simulink model "a_T_vector"  (R2016b)
settings: Solver=VariableStepAuto  StartTime=0.0  StopTime=tgoest  RelTol=1e-3
values from neighbouring files (symbols this model uses):
  m0 = 58000    [E_Guidance_Modular.m]    (also in E_Guidance_Wong.m; E_Guidance_advanced.m; E_Guidance_advanced_hybrid.m; E_Guidance_advanced_thrust_optimization.m)
  mu = 4.282828185603917*10^13    (= 4.2828281856e+13)    [E_Guidance_Modular.m]    (also in E_Guidance_Wong.m; E_Guidance_advanced.m; E_Guidance_advanced_hybrid.m; E_Guidance_advanced_thrust_optimization.m)
  r0 = A*r0    [E_Guidance_Modular.m]    (also in E_Guidance_Wong.m; E_Guidance_advanced.m; E_Guidance_advanced_hybrid.m; E_Guidance_advanced_thrust_optimization.m)
  rf = A*rf    [E_Guidance_Modular.m]    (also in E_Guidance_Wong.m; E_Guidance_advanced.m; E_Guidance_advanced_hybrid.m; E_Guidance_advanced_thrust_optimization.m)
  T_max = 800000    [E_Guidance_Modular.m]    (also in E_Guidance_Wong.m; E_Guidance_advanced.m; E_Guidance_advanced_hybrid.m; E_Guidance_advanced_thrust_optimization.m)
  T_min = 200000    [E_Guidance_Modular.m]    (also in E_Guidance_Wong.m; E_Guidance_advanced.m; E_Guidance_advanced_hybrid.m; E_Guidance_advanced_thrust_optimization.m)
  tgoest = 70    [E_Guidance_sim.m]
  V0 = A*V0    [E_Guidance_Modular.m]    (also in E_Guidance_Wong.m; E_Guidance_advanced.m; E_Guidance_advanced_hybrid.m; E_Guidance_advanced_thrust_optimization.m)
  v_ex = 3531.7    [E_Guidance_Modular.m]    (also in E_Guidance_Wong.m; E_Guidance_advanced.m; E_Guidance_advanced_hybrid.m; E_Guidance_advanced_thrust_optimization.m)
  Vf = A*Vf    [E_Guidance_Modular.m]    (also in E_Guidance_Wong.m; E_Guidance_advanced.m; E_Guidance_advanced_hybrid.m; E_Guidance_advanced_thrust_optimization.m)
settings Model: Creator=lloyd.strohl  LastModifiedBy=lloyd.strohl

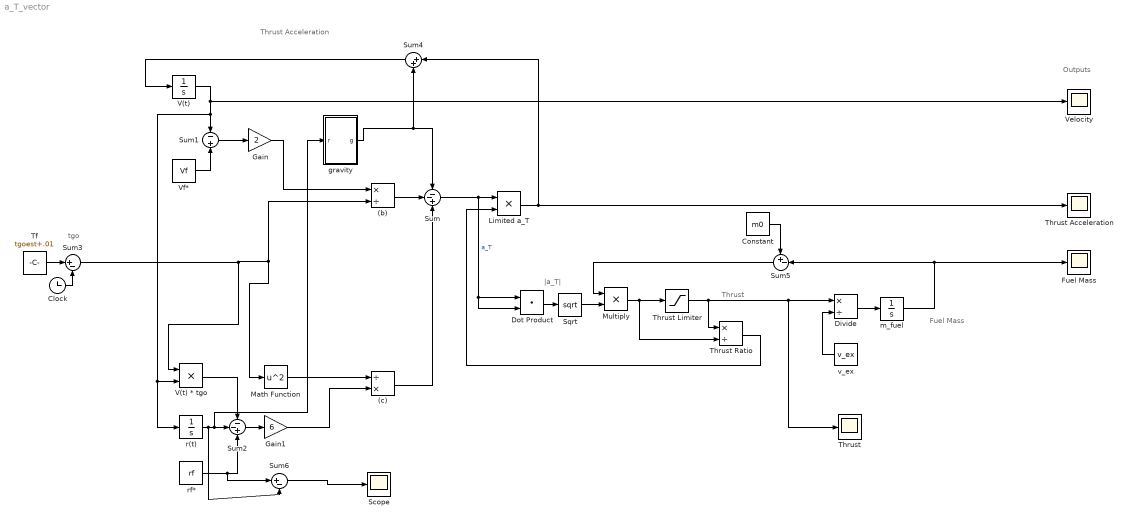
== system a_T_vector ==
  note: Thrust
  note: Fuel Mass
  note: Outputs
  note: Thrust Acceleration
  note: |a_T|
  note: tgo
  (b) : Product  Inputs=*/
  (c) : Product  Inputs=/*
  Clock : Clock
  Constant : Constant  Value=m0
  Divide : Product  Inputs=*/
  Dot Product : DotProduct  InputSameDT=on  OutDataTypeStr=Inherit: Inherit via internal rule
  Fuel Mass : Scope
  Gain : Gain  Gain=2
  Gain1 : Gain  Gain=6
  Limited a_T : Product  Inputs=**
  Math Function : Math  Operator=square  SaturateOnIntegerOverflow=on
  Multiply : Product
  Scope : Scope
  Sqrt : Sqrt  SaturateOnIntegerOverflow=on
  Sum : Sum  Inputs=--+
  Sum1 : Sum  Inputs=-+
  Sum2 : Sum  Inputs=--+
  Sum3 : Sum  Inputs=|+-
  Sum4 : Sum  Inputs=|++
  Sum5 : Sum  Inputs=+-|
  Sum6 : Sum  Inputs=|+-
  Tf : Constant  Value=tgoest+.01
  Thrust : Scope
  Thrust Acceleration : Scope
  Thrust Limiter : Saturate  UpperLimit=T_max  LowerLimit=T_min
  Thrust Ratio : Product  Inputs=*/
  V(t) : Integrator  InitialCondition=V0
  V(t) * tgo : Product
  Velocity : Scope
  Vf* : Constant  Value=Vf
  gravity : Subsystem
  m_fuel : Integrator
  r(t) : Integrator  InitialCondition=r0
  rf* : Constant  Value=rf
  v_ex : Constant  Value=v_ex
  wires:
  r(t)/1 -> Sum6/2, gravity/1(r), Sum2/2
  Tf/1 -> Sum3/1
  Clock/1 -> Sum3/2
  V(t)/1 -> Sum1/1, V(t) * tgo/2, r(t)/1, Velocity/1
  (b)/1 -> Sum/2
  Sum1/1 -> Gain/1
  Gain/1 -> (b)/1
  Sum2/1 -> Gain1/1
  Gain1/1 -> (c)/2
  Sum3/1 -> Math Function/1, (b)/2, V(t) * tgo/1
  Math Function/1 -> (c)/1
  (c)/1 -> Sum/3
  rf*/1 -> Sum6/1, Sum2/3
  V(t) * tgo/1 -> Sum2/1
  Vf*/1 -> Sum1/2
  Sqrt/1 -> Multiply/2
  v_ex/1 -> Divide/2
  Divide/1 -> m_fuel/1
  m_fuel/1 -> Sum5/2, Fuel Mass/1
  Sum4/1 -> V(t)/1
  Sum5/1 -> Multiply/1
  Constant/1 -> Sum5/1
  Dot Product/1 -> Sqrt/1
  Multiply/1 -> Thrust Ratio/2, Thrust Limiter/1
  Thrust Limiter/1 -> Thrust Ratio/1, Thrust/1, Divide/1
  Sum/1 -> Dot Product/2, Dot Product/1, Limited a_T/1  "a_T"
  Thrust Ratio/1 -> Limited a_T/2
  Limited a_T/1 -> Sum4/1, Thrust Acceleration/1
  gravity/1(g) -> Sum4/2, Sum/1
  Sum6/1 -> Scope/1

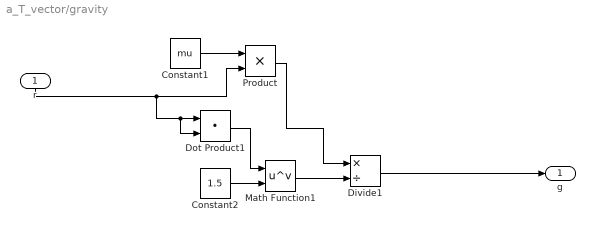
== system a_T_vector/gravity ==
  r : Inport
  Constant1 : Constant  Value=mu
  Constant2 : Constant  Value=1.5
  Divide1 : Product  Inputs=*/
  Dot Product1 : DotProduct  InputSameDT=on  OutDataTypeStr=Inherit: Inherit via internal rule
  Math Function1 : Math  Operator=pow  SaturateOnIntegerOverflow=on
  Product : Product
  g : Outport
  wires:
  r/1 -> Product/2, Dot Product1/2, Dot Product1/1
  Math Function1/1 -> Divide1/2
  Product/1 -> Divide1/1
  Constant2/1 -> Math Function1/2
  Constant1/1 -> Product/1
  Dot Product1/1 -> Math Function1/1
  Divide1/1 -> g/1
